simulink model "FastMarchingFL3Model"  (Simulink 6.6)
settings: Solver=FixedStepDiscrete  StartTime=0.0  StopTime=0  FixedStep=0.1  RelTol=1e-3
libraries: SimITKLibraryFL3 x7
settings Model: Creator=3kml  LastModifiedBy=3kml

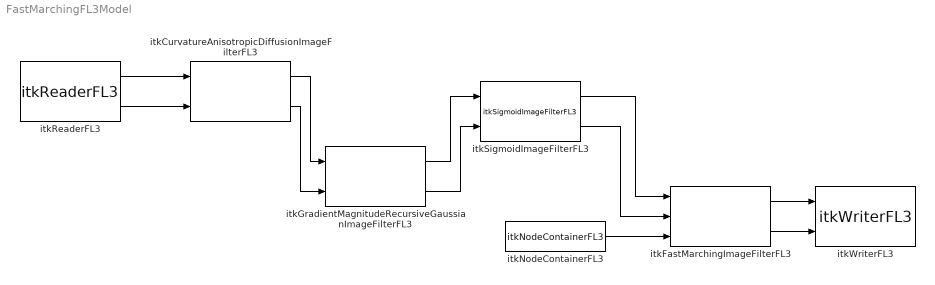
== system FastMarchingFL3Model ==
  itkCurvatureAnisotropicDiffusionImageFilterFL3 : SimITKLibraryFL3/itkCurvatureAnisotropicDiffusionImageFilterFL3  ConductanceParameter=9.0  NumberOfIterations=5  TimeStep=0.0625
  itkFastMarchingImageFilterFL3 : SimITKLibraryFL3/itkFastMarchingImageFilterFL3  StoppingValue=100
  itkGradientMagnitudeRecursiveGaussianImageFilterFL3 : SimITKLibraryFL3/itkGradientMagnitudeRecursiveGaussianImageFilterFL3  Sigma=1.0
  itkNodeContainerFL3 : SimITKLibraryFL3/itkNodeContainerFL3  Value=[0.5]  Index=[101 118 98]
  itkReaderFL3 : SimITKLibraryFL3/itkReaderFL3  FileName='subject04_t1w_p4_float.mha'
  itkSigmoidImageFilterFL3 : SimITKLibraryFL3/itkSigmoidImageFilterFL3  Alpha=-15  Beta=2.0  OutputMaximum=1  OutputMinimum=0
  itkWriterFL3 : SimITKLibraryFL3/itkWriterFL3  FileName='outputFastMarchingFL3Model.mhd'
  wires:
  itkReaderFL3/1 -> itkCurvatureAnisotropicDiffusionImageFilterFL3/1
  itkReaderFL3/2 -> itkCurvatureAnisotropicDiffusionImageFilterFL3/2
  itkGradientMagnitudeRecursiveGaussianImageFilterFL3/1 -> itkSigmoidImageFilterFL3/1
  itkGradientMagnitudeRecursiveGaussianImageFilterFL3/2 -> itkSigmoidImageFilterFL3/2
  itkSigmoidImageFilterFL3/1 -> itkFastMarchingImageFilterFL3/1
  itkSigmoidImageFilterFL3/2 -> itkFastMarchingImageFilterFL3/2
  itkFastMarchingImageFilterFL3/1 -> itkWriterFL3/1
  itkFastMarchingImageFilterFL3/2 -> itkWriterFL3/2
  itkNodeContainerFL3/1 -> itkFastMarchingImageFilterFL3/3
  itkCurvatureAnisotropicDiffusionImageFilterFL3/1 -> itkGradientMagnitudeRecursiveGaussianImageFilterFL3/1
  itkCurvatureAnisotropicDiffusionImageFilterFL3/2 -> itkGradientMagnitudeRecursiveGaussianImageFilterFL3/2
